simulink model "simulink_test"  (R2024b)
settings: Solver=VariableStepAuto  StartTime=0.0  StopTime=100  RelTol=1e-3
model workspace (MAT data in the model file):
  T = [-0.009 0.151 -1.04 4.149 -39.9326 82.2813 0.1843]
undefined symbols (not defined in the file or in its folder): daq
libraries: daqlib x1
settings Model: Creator=User  LastModifiedBy=User

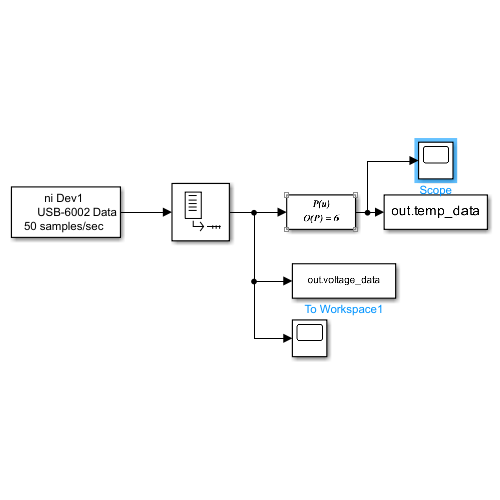
[thumbnail: Simulink's stored preview of the top-level diagram]
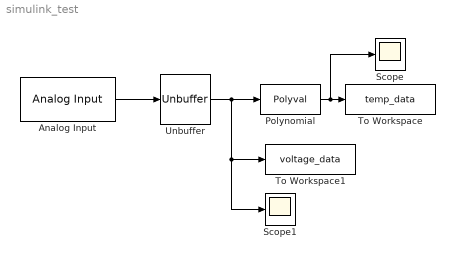
== system simulink_test ==
  Analog Input : daqlib/Analog Input  DeviceMenu=ni Dev1 (USB-6002)  Device=ni Dev1 (USB-6002)  ObjConstructor=daq.createSession('ni')  NChannelsSelected=1  Channels=1$ai0$$Dev1$1$1$2$1$#0$ai1$$Dev1$1$1$2$1$#0$ai2$$Dev1$1$1$2$1$#0$ai3$$Dev1$1$1$2$1$#0$ai4$$Dev1$1$1$1$1$#0$ai5$$Dev1$1$1$1$1$#0$ai6$$Dev1$1$1$1$1$#0$ai7$$Dev1$1$1$1$1$#  NPorts=1 for all channels  SampleRate=50  ActualRate=50  ScansPerTrigger=50  OutputTimestamp=off  AcqMode=0  NumFrameBuffer=100  OutputTriggertime=off
  Polynomial : Polyval  Coefs=T
  Scope : Scope
  Scope1 : Scope
  To Workspace : ToWorkspace  VariableName=temp_data  SaveFormat=Timeseries  SampleTime=-1
  To Workspace1 : ToWorkspace  VariableName=voltage_data  SaveFormat=Timeseries  SampleTime=-1
  Unbuffer : Unbuffer
  wires:
  Polynomial/1 -> Scope/1, To Workspace/1
  Analog Input/1 -> Unbuffer/1
  Unbuffer/1 -> Scope1/1, To Workspace1/1, Polynomial/1
